simulink model "houseHeat_model"  (R2023b)
settings: Solver=VariableStepAuto  StartTime=0.0  StopTime=24  FixedStep=1  RelTol=1e-3  EnableMultiTasking=on
undefined symbols (not defined in the file or in its folder): DiscIntNeverNeededParam, Tmax, Tmin
libraries: simulink x4, rllib x1
settings Model: Creator=The MathWorks, Inc.  LastModifiedBy=hdt
settings SolverCC: AlgebraicLoopSolver=TrustRegion  MinimalZcImpactIntegration=on
settings DataIOCC: LimitDataPoints=on  SaveFormat=Array  ReturnWorkspaceOutputs=off
settings OptimizationCC: ReuseModelBlockBuffer=off  LifeSpan=inf
settings DebuggingCC: UnconnectedInputMsg=warning  UnconnectedOutputMsg=warning  UnconnectedLineMsg=warning  SFUnexpectedBacktrackingDiag=warning  SFNoUnconditionalDefaultTransitionDiag=warning  SFExecutionAtInitializationDiag=none  ArithmeticOperatorsInVariantConditions=warning
settings HardwareCC: ProdBitPerPointer=32  ProdBitPerSizeT=32  ProdBitPerPtrDiffT=32  ProdLargestAtomicFloat=None  ProdIntDivRoundTo=Undefined  ProdEndianess=Unspecified  ProdWordSize=32  ProdHWDeviceType=32-bit Generic
settings ModelReferenceCC: EnableRefExpFcnMdlSchedulingChecks=on  PropagateSignalLabelsOutOfModel=off
settings SFSimCC: SimUseLocalCustomCode=off  CustomCodeUndefinedFunction=UseInterfaceOnly
settings RTWCC: RTWUseLocalCustomCode=off
settings CodeAppCC: StateflowObjectComments=on
settings GRTTargetCC: TargetLangStandard=C89/C90 (ANSI)
settings ConfigComp: CovMetricSettings=dw  CovSaveCumulativeToWorkspaceVar=on  CovSaveSingleToWorkspaceVar=on  CovExternalEMLEnable=off  CovSFcnEnable=off

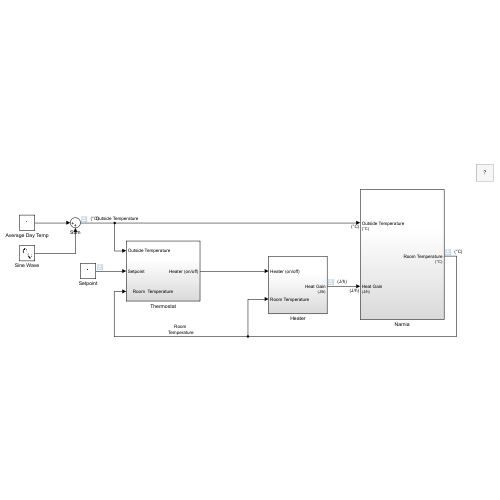
[thumbnail: Simulink's stored preview of the top-level diagram]
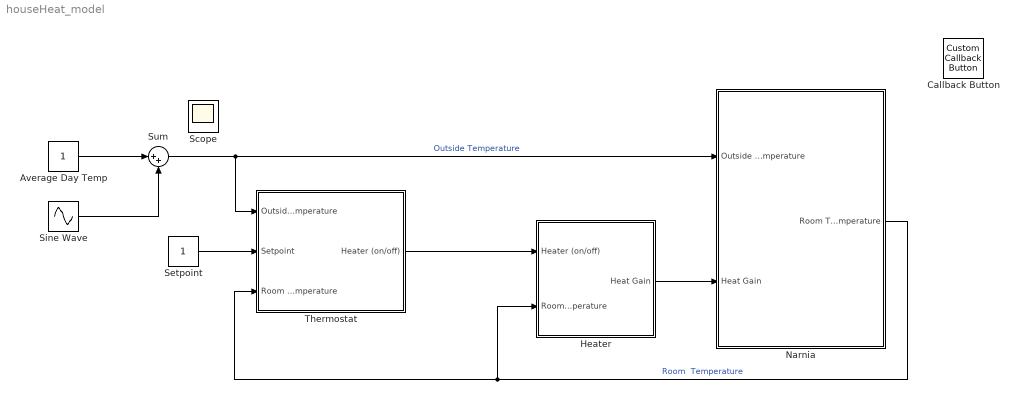
== system houseHeat_model ==
  Average Day Temp : Constant
  Callback Button : CustomCallbackButton  Configuration="{\"components\":[{\"name\":\"BackgroundImageComponent\",\"settings\":{\"image\":{\"size\":[0,0],\"src\":\"default\",\"srcOrientation\":\"Right\"},\"position\":[0,0,1,1]}},{\"name\":\"ButtonStateComponent\",\"settings\":{\"buttonType\":\"momentary\",\"clickFcn\":\"showExample('simulink\\/OpenCompletedHouseSystemModelExample')\",\"onValue\":1,\"position\":[0,0,1,1],\"pressDelay\":\"500\",\"pressFcn\":\"\",\"repeatInterval\":\"0\",\"states\":[{\"horizontalAlignment\":\"center\",\"image\":{\"position\":[0,0,1,1],\"size\":[1,1],\"src\":\"default\",\"srcOrientation\":\"Right\"},\"label\":{\"color\":[0.01176470588,0.01176470588,0.01176470588,1],\"icon\":{\"size\":[0,0],\"src\":\"default\",\"srcOrientation\":\"Right\"},\"iconPlacement\":\"left\",\"opacity\":1,\"show\":true,\"text\":{\"content\":\"?\",\"font\":\"Helvetica\",\"fontSize\":14.735309999999998}},\"labelOffset\":[0,0],\"verticalAlignment\":\"middle\"},{\"horizontalAlignment\":\"center\",\"image\":{\"position\":[0,0,1,1],\"size\":[1,1],\"src\":\"default\",\"srcOrientation\":\"Right\"},\"label\":{\"color\":[0.01176470588,0.01176470588,0.01176470588,1],\"icon\":{\"size\":[0,0],\"src\":\"default\",\"srcOrientation\":\"Right\"},\"iconPlacement\":\"left\",\"opacity\":1,\"show\":true,\"text\":{\"content\":\"?\",\"font\":\"Helvetica\",\"fontSize\":14.735309999999998}},\"labelOffset\":[0,0],\"verticalAlignment\":\"middle\"},{\"horizontalAlignment\":\"center\",\"image\":{\"position\":[0,0,1,1],\"size\":[1,1],\"src\":\"default\",\"srcOrientation\":\"Right\"},\"label\":{\"color\":[0.01176470588,0.01176470588,0.01176470588,1],\"icon\":{\"size\":[0,0],\"src\":\"default\",\"srcOrientation\":\"Right\"},\"iconPlacement\":\"left\",\"opacity\":1,\"show\":true,\"text\":{\"content\":\"?\",\"font\":\"Helvetica\",\"fontSize\":14.735309999999998}},\"labelOffset\":[0,0],\"verticalAlignment\":\"middle\"},{\"horizontalAlignment\":\"center\",\"image\":{\"position\":[0,0,1,1],\"size\":[1,1],\"src\":\"default\",\"srcOrientation\":\"Right\"},\"label\":{\"color\":[0.01176470588,0.01176470588,0.01176470588,1],\"icon\":{\"size\":[0,0],\"src\":\"default\",\"srcOrientation\":\"Right\"},\"iconPlacement\":\"left\",\"opacity\":1,\"show\":true,\"text\":{\"content\":\"?\",\"font\":\"Helvetica\",\"fontSize\":14.735309999999998}},\"labelOffset\":[0,0],\"verticalAlignment\":\"middle\"}]}},{\"name\":\"ForegroundImageComponent\",\"settings\":{\"image\":{\"size\":[0,0],\"src\":\"default\",\"srcOrientation\":\"Right\"},\"isForeground\":1,\"position\":[0,0,1,1]}}],\"settings\":{\"BindingType\":\"standalone\",\"backgroundColor\":[244,244,244,1],\"backgroundOffset\":0,\"backgroundOpacity\":1,\"fixedAspectRatio\":\"off\",\"foregroundColor\":[0.01176470588,0.01176470588,0.01176470588,1],\"migratedFromLegacy\":true,\"useBackgroundColor\":true,\"variant\":\"callback\",\"version\":\"R2023a\"},\"type\":\"Button\"}"  CustomBackgroundColor="{\"color\":[0.9568627451,0.9568627451,0.9568627451],\"show\":true}"
  Heater : Subsystem
  Narnia : Subsystem
  Setpoint : Constant
  Sine Wave : Sin  Amplitude=8  Frequency=2*pi/(3600*24)  SampleTime=600
  Sum : Sum  Inputs=|++
  Thermostat : Subsystem
  Scope : Scope
  wires:
  Thermostat/1(Heater (on/off)) -> Heater/1(Heater (on/off))
  Heater/1(Heat Gain) -> Narnia/2("Heat Gain ")
  Narnia/1(Room Temperature) -> Heater/2(Room Temperature), Thermostat/3("    Room Temperature")  "Room  Temperature"
  Setpoint/1 -> Thermostat/2(Setpoint)
  Sum/1 -> Thermostat/1(Outside Temperature), Narnia/1(Outside Temperature)  "Outside Temperature"
  Sine Wave/1 -> Sum/2
  Average Day Temp/1 -> Sum/1

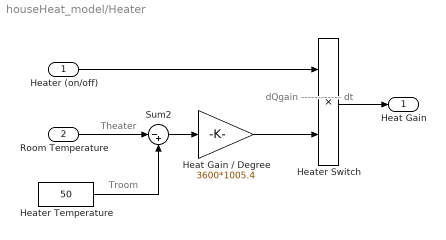
== system houseHeat_model/Heater ==
  note: dQgain
      | ------------
      |    dt
  note: Troom
  note: Theater
  Heater (on/off) : Inport
  Room Temperature : Inport  Port=2
  Heat Gain / Degree : Gain  Gain=3600*1005.4
  Heater Switch : Product  RndMeth=Zero
  Heater Temperature : Constant  Value=50
  Sum2 : Sum  Inputs=|-+
  Heat Gain : Outport  Unit=joule/hour  VectorParamsAs1DForOutWhenUnconnected=off
  wires:
  Heater Temperature/1 -> Sum2/2
  Room Temperature/1 -> Sum2/1
  Sum2/1 -> Heat Gain / Degree/1
  Heat Gain / Degree/1 -> Heater Switch/2
  Heater (on/off)/1 -> Heater Switch/1
  Heater Switch/1 -> Heat Gain/1

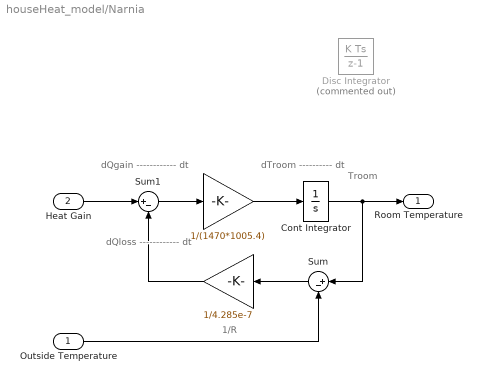
== system houseHeat_model/Narnia ==
  note: 1/R
  note: Troom
  note: dQloss
      | ------------
      |      dt
  note: dQgain
      | ------------
      |      dt
  note: dTroom
      | ----------
      |     dt
  Outside Temperature : Inport  Unit=°C
  "Heat Gain " : Inport  Port=2  Unit=joule/h
  " " : Gain  Gain=1/4.285e-7  SaturateOnIntegerOverflow=on  OutDataTypeStr=Inherit: Same as input  ParamDataTypeStr=Inherit: Same as input
  "  " : Gain  Gain=1/(1470*1005.4)  SaturateOnIntegerOverflow=on  OutDataTypeStr=Inherit: Same as input  ParamDataTypeStr=Inherit: Same as input
  Cont Integrator : Integrator  InitialCondition=20
  Disc Integrator : DiscreteIntegrator  Commented=on  SampleTime=-1  ICPrevOutput=DiscIntNeverNeededParam  ICPrevScaledInput=DiscIntNeverNeededParam
  Sum : Sum  Inputs=|+-
  Sum1 : Sum  Inputs=|+-  InputSameDT=on  SaturateOnIntegerOverflow=on  OutDataTypeStr=Inherit: Same as first input
  Room Temperature : Outport  Unit=°C  VectorParamsAs1DForOutWhenUnconnected=off
  wires:
  "Heat Gain "/1 -> Sum1/1
  Sum1/1 -> "  "/1
  "  "/1 -> Cont Integrator/1
  Cont Integrator/1 -> Room Temperature/1, Sum/1
  " "/1 -> Sum1/2
  Sum/1 -> " "/1
  Outside Temperature/1 -> Sum/2

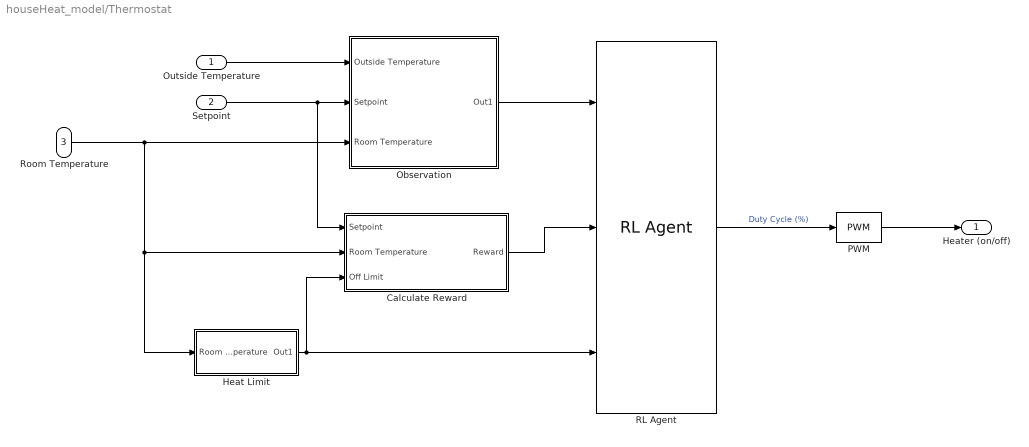
== system houseHeat_model/Thermostat ==
  Outside Temperature : Inport
  Setpoint : Inport  Port=2
  "    Room Temperature" : Inport  Port=3
  Calculate Reward : Subsystem
  Heat Limit : Subsystem
  Observation : Subsystem
  PWM : simulink/Discontinuities/PWM  DisableCoverage=on  Period=600  InitialDelay=0  DisallowZeroDutyCycle=off  RunAtFixedTimeIntervals=off  SampleTime=0.1
  RL Agent : rllib/RL Agent  Agent=agent  ExternalActionAsInput=off  ProvideLastAction=off  ProvideCumRwd=off  TreatAsDirectFeedthrough=on  UseStrictObservationDataTypes=off
  Heater (on/off) : Outport  VectorParamsAs1DForOutWhenUnconnected=off
  wires:
  Setpoint/1 -> Calculate Reward/1(Setpoint), Observation/2(Setpoint)
  "    Room Temperature"/1 -> Observation/3("    Room Temperature"), Heat Limit/1("    Room Temperature"), Calculate Reward/2("    Room Temperature")
  Outside Temperature/1 -> Observation/1(Outside Temperature)
  Observation/1(Out1) -> RL Agent/1
  Calculate Reward/1(Reward) -> RL Agent/2
  Heat Limit/1(Out1) -> Calculate Reward/3(Off Limit), RL Agent/3
  RL Agent/1 -> PWM/1  "Duty Cycle (%)"
  PWM/1 -> Heater (on/off)/1

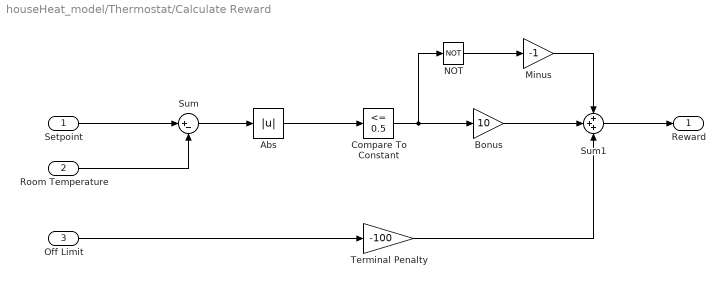
== system houseHeat_model/Thermostat/Calculate Reward ==
  Setpoint : Inport
  "    Room Temperature" : Inport  Port=2
  Off Limit : Inport  Port=3
  Abs : Abs  SaturateOnIntegerOverflow=off
  Bonus : Gain  Gain=10
  Compare To Constant : simulink/Logic and Bit Operations/Compare To Constant  relop=<=  const=0.5  OutDataTypeStr=boolean
  Minus : Gain  Gain=-1
  NOT : Logic  Operator=NOT  IconShape=distinctive  AllPortsSameDT=off  OutDataTypeStr=boolean
  Sum : Sum  Inputs=|+-
  Sum1 : Sum  Inputs=+++
  Terminal Penalty : Gain  Gain=-100
  Reward : Outport
  wires:
  Setpoint/1 -> Sum/1
  "    Room Temperature"/1 -> Sum/2
  Sum/1 -> Abs/1
  Abs/1 -> Compare To Constant/1
  NOT/1 -> Minus/1
  Compare To Constant/1 -> Bonus/1, NOT/1
  Bonus/1 -> Sum1/2
  Minus/1 -> Sum1/1
  Sum1/1 -> Reward/1
  Terminal Penalty/1 -> Sum1/3
  Off Limit/1 -> Terminal Penalty/1

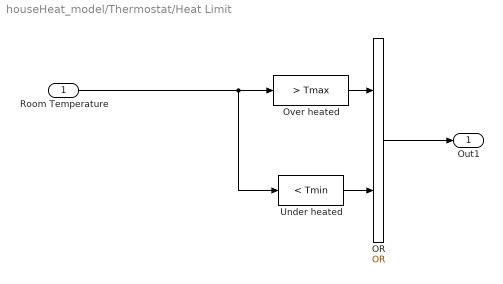
== system houseHeat_model/Thermostat/Heat Limit ==
  "    Room Temperature" : Inport
  OR : Logic  Operator=OR  IconShape=distinctive  AllPortsSameDT=off  OutDataTypeStr=boolean
  Over heated : simulink/Logic and Bit Operations/Compare To Constant  relop=>  const=Tmax  OutDataTypeStr=boolean
  Under heated : simulink/Logic and Bit Operations/Compare To Constant  relop=<  const=Tmin  OutDataTypeStr=boolean
  Out1 : Outport
  wires:
  "    Room Temperature"/1 -> Under heated/1, Over heated/1
  Under heated/1 -> OR/2
  Over heated/1 -> OR/1
  OR/1 -> Out1/1

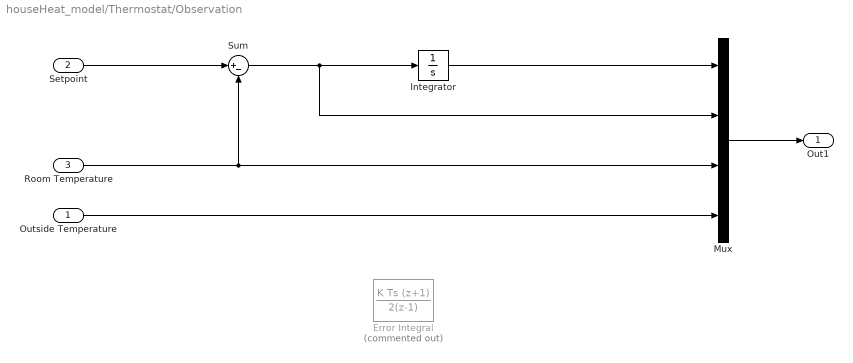
== system houseHeat_model/Thermostat/Observation ==
  Outside Temperature : Inport
  Setpoint : Inport  Port=2
  "    Room Temperature" : Inport  Port=3
  Error Integral : DiscreteIntegrator  Commented=on  IntegratorMethod=Integration: Trapezoidal  SampleTime=600  ICPrevOutput=DiscIntNeverNeededParam  ICPrevScaledInput=DiscIntNeverNeededParam
  Integrator : Integrator
  Mux : Mux
  Sum : Sum  Inputs=|+-
  Out1 : Outport
  wires:
  Outside Temperature/1 -> Mux/4
  Setpoint/1 -> Sum/1
  "    Room Temperature"/1 -> Sum/2, Mux/3
  Sum/1 -> Integrator/1, Mux/2
  Integrator/1 -> Mux/1
  Mux/1 -> Out1/1
